simulink model "Example_Unknown_Input_Observer_Simulink"  (Simulink 9.0)
settings: Solver=FixedStepAuto  StartTime=0.0  StopTime=20  FixedStep=1e-3  RelTol=1e-3  EnableMultiTasking=on
settings Model: SuppressorTable=22 serialization::archive 11 0 6 0 0 0 0 0  Creator=Pierre-Marie.Damon  LastModifiedBy=PierreMarieDamon
settings DataIOCC: SaveFormat=Dataset
settings DebuggingCC: UnderspecifiedInitializationDetection=Simplified  MergeDetectMultiDrivingBlocksExec=error
settings HardwareCC: ProdBitPerPointer=64  ProdBitPerSizeT=64  ProdBitPerPtrDiffT=64  ProdLargestAtomicFloat=Float  ProdIntDivRoundTo=Zero  ProdEndianess=LittleEndian  ProdWordSize=64  ProdHWDeviceType=Intel->x86-64 (Windows64)
settings ModelReferenceCC: PropagateSignalLabelsOutOfModel=on
settings GRTTargetCC: GeneratePreprocessorConditionals=Disable all

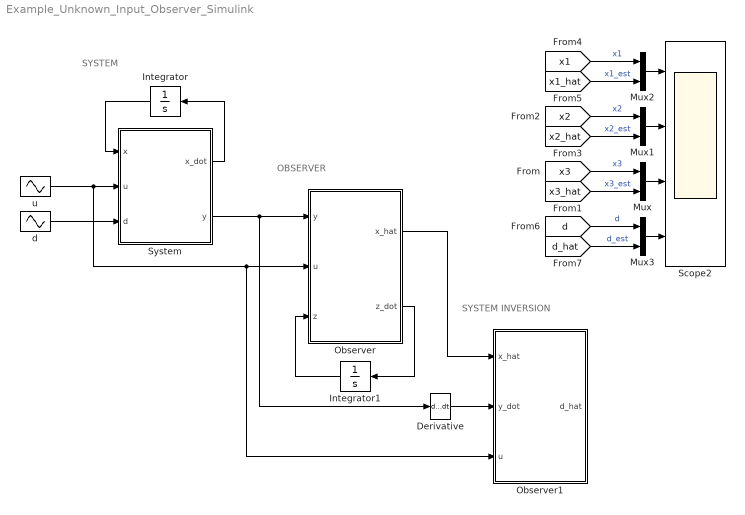
== system Example_Unknown_Input_Observer_Simulink ==
  note: OBSERVER
  note: SYSTEM
  note: SYSTEM INVERSION
  Derivative : Derivative
  Integrator : Integrator  InitialCondition=[1 0 2]
  Integrator1 : Integrator  InitialCondition=[0 0 0]
  Mux{,1..3} (4 alike) : Mux  Inputs=2
  Observer : Subsystem
  Observer1 : Subsystem
  Scope2 : Scope  NumInputPorts=4
  System : Subsystem
  d : Sin  Amplitude=0.5  Frequency=10  SampleTime=0
  u : Sin  SampleTime=0
  wires:
  u/1 -> System/2(u), Observer1/3("u "), Observer/2(u)
  System/1(x_dot) -> Integrator/1
  Integrator/1 -> System/1(x)
  System/2(y) -> Derivative/1, Observer/1(y)
  Observer/2(z_dot) -> Integrator1/1
  Integrator1/1 -> Observer/3(z)
  [x3] -> Mux/1  "x3"
  [x3_hat] -> Mux/2  "x3_est"
  Mux/1 -> Scope2/3
  d/1 -> System/3(d)
  [x2] -> Mux1/1  "x2"
  [x2_hat] -> Mux1/2  "x2_est"
  Mux1/1 -> Scope2/2
  [x1] -> Mux2/1  "x1"
  [x1_hat] -> Mux2/2  "x1_est"
  Mux2/1 -> Scope2/1
  Observer/1(x_hat) -> Observer1/1("x_hat ")
  Derivative/1 -> Observer1/2(y_dot)
  Mux3/1 -> Scope2/4
  [d_hat] -> Mux3/2  "d_est"
  [d] -> Mux3/1  "d"

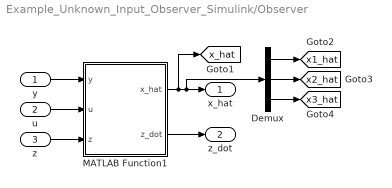
== system Example_Unknown_Input_Observer_Simulink/Observer ==
  y : Inport
  u : Inport  Port=2
  z : Inport  Port=3
  Demux : Demux  Outputs=3
  MATLAB Function1 : MATLAB Function  TreatAsAtomicUnit=on
  x_hat : Outport
  z_dot : Outport  Port=2
  tag scope: x1_hat=global, x2_hat=global, x3_hat=global, x_hat=global
  wires:
  MATLAB Function1/1(x_hat) -> [x_hat], Demux/1, x_hat/1
  y/1 -> MATLAB Function1/1(y)
  MATLAB Function1/2(z_dot) -> z_dot/1
  u/1 -> MATLAB Function1/2(u)
  z/1 -> MATLAB Function1/3(z)
  Demux/1 -> [x1_hat]
  Demux/2 -> [x2_hat]
  Demux/3 -> [x3_hat]

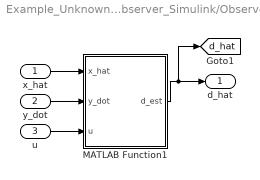
== system Example_Unknown_Input_Observer_Simulink/Observer1 ==
  "x_hat " : Inport
  y_dot : Inport  Port=2
  "u " : Inport  Port=3
  MATLAB Function1 : MATLAB Function  TreatAsAtomicUnit=on
  d_hat : Outport
  tag scope: d_hat=global
  wires:
  MATLAB Function1/1(d_est) -> [d_hat], d_hat/1
  "x_hat "/1 -> MATLAB Function1/1(x_hat)
  y_dot/1 -> MATLAB Function1/2(y_dot)
  "u "/1 -> MATLAB Function1/3(u)

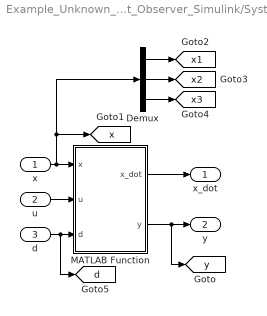
== system Example_Unknown_Input_Observer_Simulink/System ==
  x : Inport
  u : Inport  Port=2
  d : Inport  Port=3
  Demux : Demux  Outputs=3
  MATLAB Function : MATLAB Function  TreatAsAtomicUnit=on
  x_dot : Outport
  y : Outport  Port=2
  tag scope: d=global, x1=global, x2=global, x3=global, x=global, y=global
  wires:
  u/1 -> MATLAB Function/2(u)
  MATLAB Function/2(y) -> [y], y/1
  MATLAB Function/1(x_dot) -> x_dot/1
  x/1 -> Demux/1, [x], MATLAB Function/1(x)
  Demux/1 -> [x1]
  Demux/2 -> [x2]
  Demux/3 -> [x3]
  d/1 -> [d], MATLAB Function/3(d)

== matlab function Observer/MATLAB Function1 ==
  data: x_hat output double; y input double; z_dot output double; u input double; z input double
function [x_hat, z_dot]= fcn(y,u,z)

N=[	-2.0, -0.0000000000000011102230246251565404236316680908, 1.0; 
	0, -0.5, 0; 
	-2.0, 0.000000000000002664535259100375697016716003418, -8.0];


G=[	0; 
	0; 
	-1.0];


L=[	2.0; 
	0; 
	-7.0];


H=[	0; 
	-1.0; 
	-1.0];

z_dot = N*z + G*u + L*y;
x_hat = z - H*y;

== matlab function System/MATLAB Function ==
  data: x input double; x_dot output double; u input double; y output double; d input double
function [x_dot,y]= fcn(x,u,d)

A=[	-2.0, 1.0, 1.0; 
	0, -1.0, 3.0; 
	-2.0, 0, -5.0];


B=[	0; 
	1.0; 
	0];


C=[	0, 1.0, 0];


D=[	0; 
	1.0; 
	1.0];

x_dot = A*x + B*u + D*d;
y = C*x

== matlab function Observer1/MATLAB Function1 ==
  data: d_est output double; x_hat input double; y_dot input double; u input double
function d_est = fcn(x_hat,y_dot,u)
A=[	-2.0, 1.0, 1.0; 
	0, -1.0, 3.0; 
	-2.0, 0, -5.0];


B=[	0; 
	1.0; 
	0];


C=[	0, 1.0, 0];


D=[	0; 
	1.0; 
	1.0];

d_est=inv(C*D)*(y_dot-C*A*x_hat-C*B*u);
